simulink model "practicauno (2)"  (R2024b)
settings: Solver=VariableStepAuto  StartTime=0.0  StopTime=10  RelTol=1e-3
InitFcn:
  | Ip=0.0079;
  | Mc=0.7031;
  | Lp=0.3302;
  | Mp=0.23;
  | Fc=0;
  | Beq=4.3;
  | g=9.81;
  | Bp=0.0024;

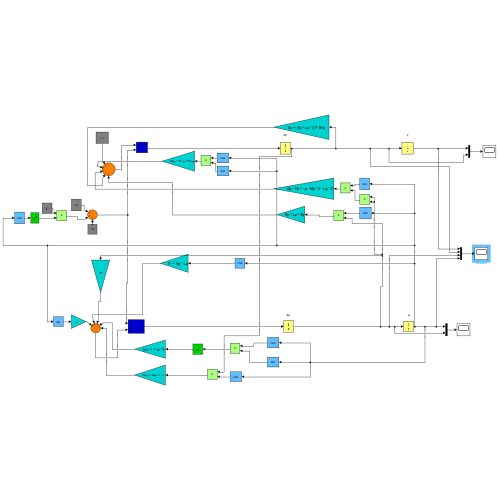
[thumbnail: Simulink's stored preview of the top-level diagram]
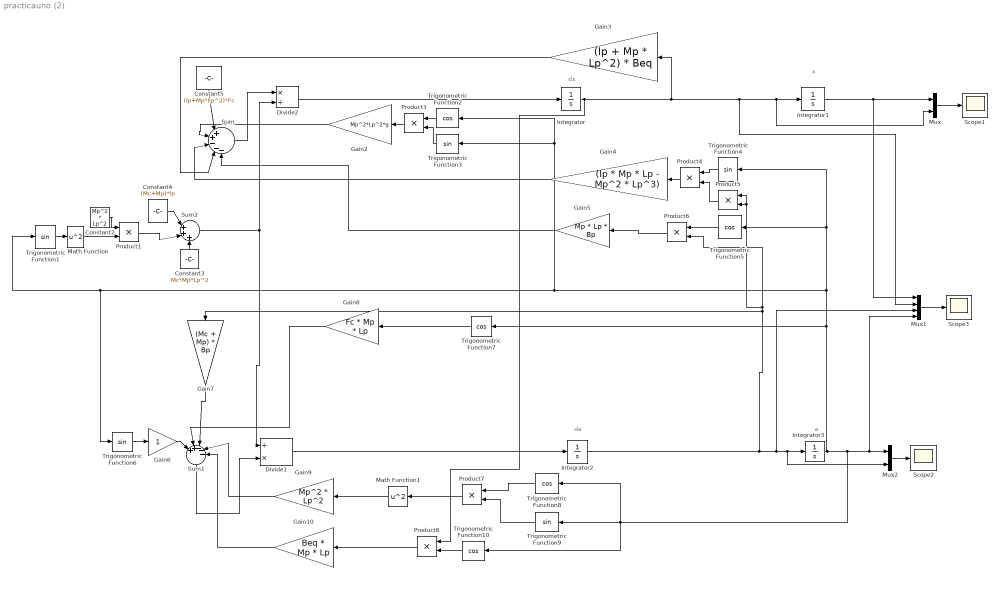
== system practicauno (2) ==
  note: x
  note: da
  note: dx
  note: a
  Constant2 : Constant  Value=Mp^2 * Lp^2
  Constant3 : Constant  Value=Mc*Mp*Lp^2
  Constant4 : Constant  Value=(Mc+Mp)*Ip
  Constant5 : Constant  Value=(Ip+Mp*Lp^2)*Fc
  Divide1 : Product  Inputs=/*
  Divide2 : Product  Inputs=*/
  Gain10 : Gain  Gain=Beq * Mp * Lp
  Gain2 : Gain  Gain=Mp^2*Lp^2*g
  Gain3 : Gain  Gain=(Ip + Mp * Lp^2) * Beq
  Gain4 : Gain  Gain=(Ip * Mp * Lp - Mp^2 * Lp^3)
  Gain5 : Gain  Gain=Mp * Lp * Bp
  Gain6 : Gain
  Gain7 : Gain  Gain=(Mc + Mp) * Bp
  Gain8 : Gain  Gain=Fc * Mp * Lp
  Gain9 : Gain  Gain=Mp^2 * Lp^2
  Integrator : Integrator
  Integrator1 : Integrator
  Integrator2 : Integrator
  Integrator3 : Integrator  InitialCondition=1 * pi/180
  Math Function : Math  Operator=square
  Math Function1 : Math  Operator=square
  Mux : Mux  Inputs=2
  Mux1 : Mux
  Mux2 : Mux  Inputs=2
  Product{1,3..8} (7 alike) : Product
  Scope1 : Scope
  Scope2 : Scope
  Scope3 : Scope
  Sum : Sum  Inputs=|++---
  Sum1 : Sum  Inputs=|++---
  Sum2 : Sum  Inputs=|+++
  Trigonometric Function{1,3..4,6,9} (5 alike) : Trigonometry
  Trigonometric Function{2,5,7..8,10} (5 alike) : Trigonometry  Operator=cos
  wires:
  Gain3/1 -> Sum/4
  Sum2/1 -> Divide1/1, Divide2/2
  Divide1/1 -> Integrator2/1
  Gain6/1 -> Sum1/1
  Trigonometric Function1/1 -> Math Function/1
  Math Function/1 -> Product1/2
  Trigonometric Function3/1 -> Product3/2
  Divide2/1 -> Integrator/1
  Trigonometric Function7/1 -> Gain8/1
  Integrator3/1 -> Mux1/4, Mux2/1, Trigonometric Function10/1, Trigonometric Function8/1, Trigonometric Function9/1, Trigonometric Function7/1, Trigonometric Function1/1, Trigonometric Function6/1, Trigonometric Function2/1, Trigonometric Function3/1, Trigonometric Function5/1, Trigonometric Function4/1
  Integrator1/1 -> Mux1/1, Mux/1
  Product4/1 -> Gain4/1
  Trigonometric Function9/1 -> Product7/2
  Math Function1/1 -> Gain9/1
  Trigonometric Function10/1 -> Product8/2
  Product3/1 -> Gain2/1
  Product1/1 -> Sum2/2
  Gain9/1 -> Sum1/4
  Trigonometric Function8/1 -> Product7/1
  Integrator/1 -> Mux1/2, Mux/2, Integrator1/1, Gain3/1, Product8/1
  Trigonometric Function4/1 -> Product4/1
  Product7/1 -> Math Function1/1
  Constant5/1 -> Sum/1
  Constant2/1 -> Product1/1
  Trigonometric Function5/1 -> Product6/1
  Sum/1 -> Divide2/1
  Trigonometric Function6/1 -> Gain6/1
  Constant3/1 -> Sum2/3
  Integrator2/1 -> Product6/2, Product5/2, Product5/1, Gain7/1, Mux1/3, Mux2/2, Integrator3/1
  Gain5/1 -> Sum/5
  Gain10/1 -> Sum1/5
  Trigonometric Function2/1 -> Product3/1
  Product6/1 -> Gain5/1
  Gain7/1 -> Sum1/3
  Gain8/1 -> Sum1/2
  Sum1/1 -> Divide1/2
  Product8/1 -> Gain10/1
  Product5/1 -> Product4/2
  Gain2/1 -> Sum/2
  Gain4/1 -> Sum/3
  Constant4/1 -> Sum2/1
  Mux/1 -> Scope1/1
  Mux2/1 -> Scope2/1
  Mux1/1 -> Scope3/1
